simulink model "ex3_a"  (R2020a)
settings: Solver=VariableStepAuto  StartTime=0.0  StopTime=10.0  RelTol=1e-3
undefined symbols (not defined in the file): qde, qe
settings Model: Creator=Tomo  LastModifiedBy=Tomo

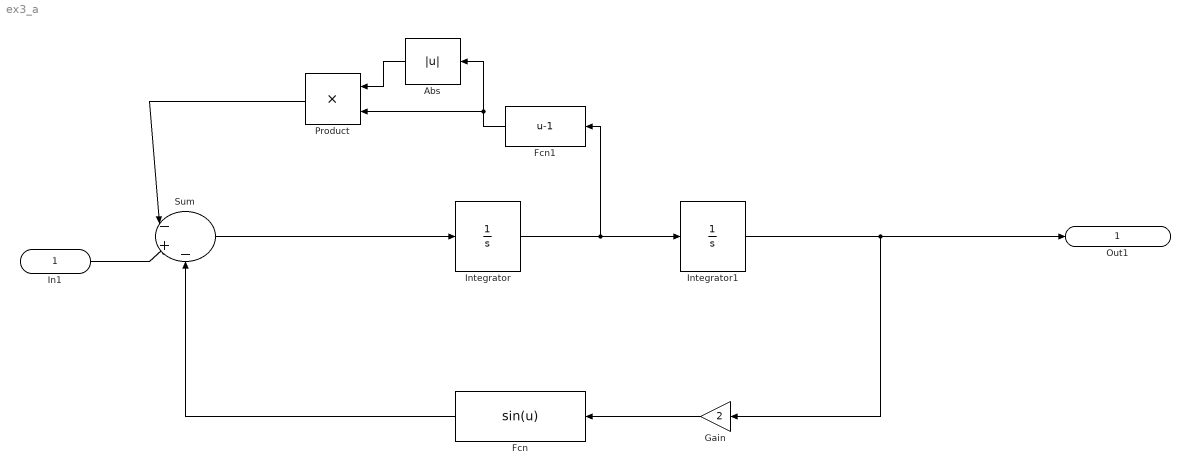
== system ex3_a ==
  In1 : Inport
  Abs : Abs
  Fcn : Fcn  Expr=sin(u)
  Fcn1 : Fcn  Expr=u-1
  Gain : Gain  Gain=2
  Integrator : Integrator  InitialCondition=qde
  Integrator1 : Integrator  InitialCondition=qe
  Product : Product
  Sum : Sum  Inputs=|-+-
  Out1 : Outport
  wires:
  Integrator1/1 -> Gain/1, Out1/1
  Integrator/1 -> Fcn1/1, Integrator1/1
  Sum/1 -> Integrator/1
  Gain/1 -> Fcn/1
  Fcn/1 -> Sum/3
  Fcn1/1 -> Product/2, Abs/1
  Abs/1 -> Product/1
  Product/1 -> Sum/1
  In1/1 -> Sum/2
